simulink model "other"  (R2025a)
settings: Solver=VariableStepAuto  StartTime=0.0  StopTime=0.1  MaxStep=1e-7  RelTol=1e-3
undefined symbols (not defined in the file): Acid, Lead
libraries: spsPWMGeneratorDCDCLib x8, spsMosfetLib x4, spsCurrentMeasurementLib x3, spsSeriesRLCBranchLib x3, spsVoltageMeasurementLib x2, spsBatteryLib x1, spsDCVoltageSourceLib x1, spsGroundLib x1, spsPVArrayLib x1, spspowerguiLib x1
settings Model: Creator=GNKRISHNAN  LastModifiedBy=GNKRISHNAN

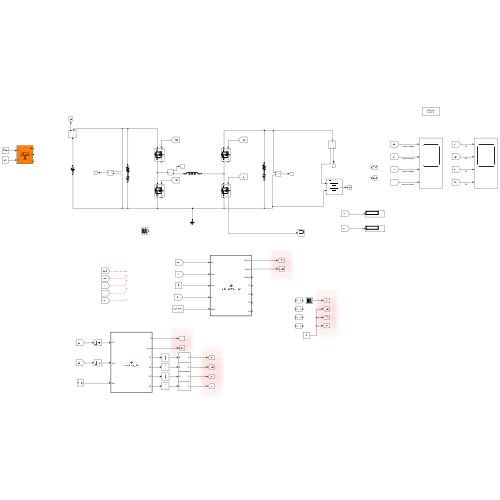
[thumbnail: Simulink's stored preview of the top-level diagram]
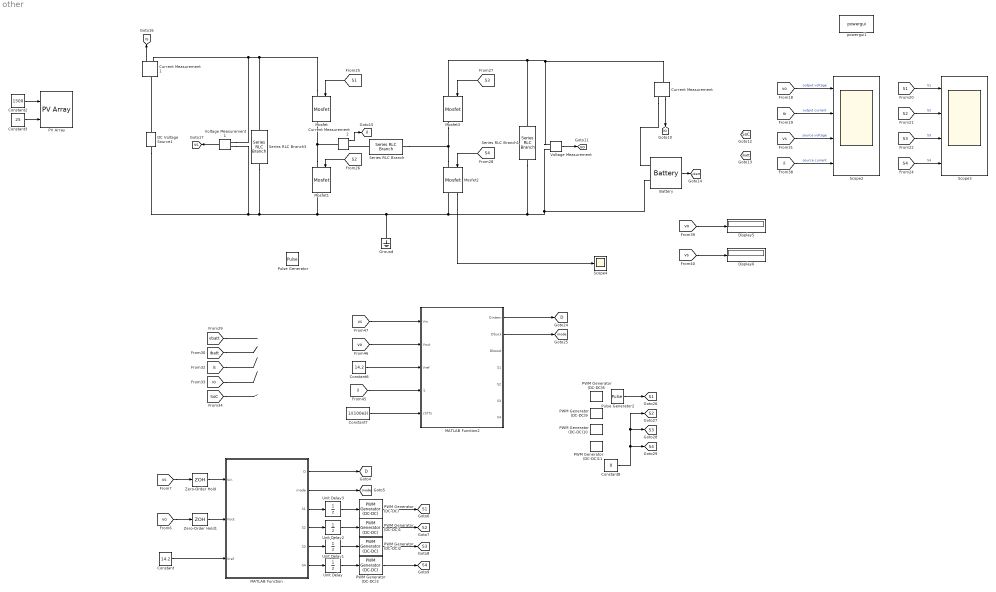
== system other ==
  Battery : spsBatteryLib/Battery  BatType=Lead-Acid  NomV=12  NomQ=5.4  SOC=80  Batt_Tr=.001  PresetModel=on  MaxQ=5.625  MinV=9  FullV=13.0658  Dis_rate=1.08  R=0.022222  Normal_OP=1.6755  expZone="[12.2171        0.018]"
  Constant : Constant  Value=14.2
  Constant2 : Constant  Value=1500
  Constant3 : Constant  Value=25
  Constant6 : Constant  Value=14.2
  Constant7 : Constant  Value=1/(100e3)
  Constant8 : Constant  Value=0
  Current Measurement : spsCurrentMeasurementLib/Current Measurement  PhasorSimulation=off  OutputType=Complex  PSBequivalent=0
  Current Measurement1 : spsCurrentMeasurementLib/Current Measurement  PhasorSimulation=off  OutputType=Complex  PSBequivalent=0
  Current Measurement2 : spsCurrentMeasurementLib/Current Measurement  PhasorSimulation=off  OutputType=Complex  PSBequivalent=0
  DC Voltage Source1 : spsDCVoltageSourceLib/DC Voltage Source  Amplitude=20  Measurements=None
  Display5 : Display
  Display6 : Display
  Ground : spsGroundLib/Ground  LConnTagsString=a
  MATLAB Function : MATLAB Function  TreatAsAtomicUnit=on  SystemSampleTime=1e-6
  MATLAB Function2 : MATLAB Function  TreatAsAtomicUnit=on  SystemSampleTime=1/(100e3)
  Mosfet{,1..3} (4 alike) : spsMosfetLib/Mosfet  Ron=0.1  Lon=0  Rd=0.0028  Vfd=0.7  IC=0  Rs=1e5  Cs=inf  Measurements=on
  PV Array : spsPVArrayLib/PV Array  Npar=1  Nser=1  PlotType=one module @ 25 deg.C & specified irradiances  S_vec="[ 1000  500  100 ]"  Temp_C_vec="[ 45 25  ]"  ModuleName=User-defined  PlotWhenSelected=off  Pm=130.032  Ncell=60  Voc=21.6  Isc=8.36  Vm=17.2  Im=7.56  beta_Voc_pc=-0.1  alpha_Isc_pc=0.001  beta_Voc=-0.0216  alpha_Isc=8.36e-05  IL=8.428  I0=1.3766e-16  nI=0.36322  Rsh=37.2573  Rs=0.33372  RobustModel=off  RobustCellTemperature=313.3991  BAL=on  Tc=1e-6  Tfilter=5e-5
  PWM Generator (DC-DC){,1..3,8..11} (8 alike) : spsPWMGeneratorDCDCLib/PWM Generator (DC-DC)  Fsw=100e3  Ts=0
  Pulse Generator : DiscretePulseGenerator  PulseType=Time based  Period=10  PulseWidth=5
  Pulse Generator2 : DiscretePulseGenerator  PulseType=Time based  Period=1/(100e3)  PulseWidth=65
  Scope2 : Scope  NumInputPorts=4
      settings: ActiveDisplayYMinimum=-3.068333797460328  ActiveDisplayYMaximum=27.615004177142961  DataLoggingVariableName=ScopeData3
  Scope3 : Scope  NumInputPorts=4
      settings: ActiveDisplayYMinimum=-0.12499999999999997  ActiveDisplayYMaximum=1.125  DataLoggingVariableName=ScopeData4
  Scope4 : Scope
      settings: ActiveDisplayYMinimum=-1.430223431644835  ActiveDisplayYMaximum=12.872010884803517  DataLoggingVariableName=ScopeData2
  Series RLC Branch : spsSeriesRLCBranchLib/Series RLC Branch  LConnTagsString=__new0  RConnTagsString=__new0  BranchType=L  Resistance=0.001  Inductance=110e-6  SetiL0=on  InitialCurrent=1  Capacitance=1e-6  Setx0=off  InitialVoltage=0  Measurements=None
  Series RLC Branch1 : spsSeriesRLCBranchLib/Series RLC Branch  LConnTagsString=__new0  RConnTagsString=__new0  BranchType=RC  Resistance=0.00001  Inductance=1e-3  SetiL0=off  InitialCurrent=0  Capacitance=120e-6  Setx0=on  InitialVoltage=12  Measurements=None
  Series RLC Branch3 : spsSeriesRLCBranchLib/Series RLC Branch  LConnTagsString=__new0  RConnTagsString=__new0  BranchType=RC  Resistance=0.0001  Inductance=1e-3  SetiL0=off  InitialCurrent=0  Capacitance=400e-6  Setx0=on  InitialVoltage=0  Measurements=None
  Unit Delay{,1..3} (4 alike) : UnitDelay  SampleTime=-1  HasFrameUpgradeWarning=on
  Voltage Measurement : spsVoltageMeasurementLib/Voltage Measurement  PhasorSimulation=off  OutputType=Complex  PSBequivalent=0
  Voltage Measurement1 : spsVoltageMeasurementLib/Voltage Measurement  PhasorSimulation=off  OutputType=Complex  PSBequivalent=0
  Zero-Order Hold : ZeroOrderHold  SampleTime=-1
  Zero-Order Hold1 : ZeroOrderHold  SampleTime=-1
  powergui1 : spspowerguiLib/powergui  Priority=1  SimulationMode=Discrete  SampleTime=1e-7  frequency=60  Iterations=50  frequencyindice=0  Pbase=100e6  ErrMax=1e-4  UnitsV=kV  UnitsW=MW  buscounter=0  FunctionMessages=off  echomessages=off  EnableUseOfTLC=off  CurrentSourceSwitches=off  DisableSnubberDevices=off  DisableRonSwitches=off  DisableVfSwitches=off  DisplayEquations=off  AutomaticDiscreteSolvers=off  SolverType=Tustin/Backward Euler (TBE)  Interpol=off  ExternalGateDelay=off  methode=off  Ts=100  x0status=blocks  SPID=on  SwTol=0  HookPort=off  NonlinearTolerance=1e-4  nMaxIteration=100  ContinueOnMaxIteration=off  RestoreLinks=warning  ResistiveCurrentMeasurement=off  Frange=[0:2:500]  Ylog=off  Xlog=on  ShowGrid=off  save=off  variable=ZData  structure=0  ZoomFFT=off  StartTime=0.0  cycles=1  DisplayStyle=1  fundamental=60  FreqAxis=off  MaxFrequency=1000  frequencyindicesteady=1  RmsSteady=1  display=off
  tag scope: D=global, S1=global, S2=global, S3=global, S4=global, SoC=global, ibatt=global, il=global, io=global, is=global, mode=global, vbatt=global, vo=global, vs=global
  wires:
  MATLAB Function/4(S2) -> Unit Delay2/1
  MATLAB Function/5(S3) -> Unit Delay1/1
  MATLAB Function/3(S1) -> Unit Delay3/1
  MATLAB Function/1(D) -> [D]
  MATLAB Function/2(mode) -> [mode]
  [vs] -> Zero-Order Hold/1
  [vo] -> Zero-Order Hold1/1
  MATLAB Function/6(S4) -> Unit Delay/1
  Constant/1 -> MATLAB Function/3(Vref)
  Zero-Order Hold/1 -> MATLAB Function/1(Vin)
  Zero-Order Hold1/1 -> MATLAB Function/2(Vout)
  PWM Generator (DC-DC)/1 -> [S1]
  PWM Generator (DC-DC)1/1 -> [S2]
  PWM Generator (DC-DC)2/1 -> [S3]
  PWM Generator (DC-DC)3/1 -> [S4]
  Unit Delay/1 -> PWM Generator (DC-DC)3/1
  Unit Delay1/1 -> PWM Generator (DC-DC)2/1
  Unit Delay2/1 -> PWM Generator (DC-DC)1/1
  Unit Delay3/1 -> PWM Generator (DC-DC)/1
  [vbatt] -> ?
  [ibatt] -> ?
  [is] -> ?
  [SoC] -> ?
  [io] -> ?
  Mosfet2/1 -> Scope4/1
  [S4] -> Scope3/4  "S4"
  [vo] -> Display5/1
  Current Measurement/1 -> [io]
  Current Measurement1/1 -> [is]
  [vs] -> Scope2/3  "source voltage"
  [S2] -> Mosfet1/1
  Voltage Measurement1/1 -> [vs]
  [S2] -> Scope3/2  "S2"
  Constant3/1 -> PV Array/2
  Voltage Measurement/1 -> [vo]
  [S1] -> Scope3/1  "S1"
  [vo] -> Scope2/1  "output voltage"
  [il] -> Scope2/4  "source current"
  [S4] -> Mosfet2/1
  [S1] -> Mosfet/1
  [S3] -> Mosfet3/1
  Current Measurement2/1 -> [il]
  [S3] -> Scope3/3  "S3"
  Battery/1 -> [vbatt]
  Constant2/1 -> PV Array/1
  [vs] -> Display6/1
  [io] -> Scope2/2  "output current"
  Constant6/1 -> MATLAB Function2/3(Vref)
  [vs] -> MATLAB Function2/1(Vin)
  MATLAB Function2/2(Dbuck) -> [mode]
  Constant7/1 -> MATLAB Function2/5(ctrlTs)
  [il] -> MATLAB Function2/4(iL)
  Pulse Generator2/1 -> [S1]
  [vo] -> MATLAB Function2/2(Vout)
  MATLAB Function2/1(Dintern) -> [D]
  Constant8/1 -> [S4], [S3], [S2]
  connections:
  Ground/LConn1 -- Mosfet1/RConn1 -- DC Voltage Source1/LConn1 -- Voltage Measurement1/LConn2 -- Series RLC Branch3/RConn1 -- Mosfet2/RConn1 -- Voltage Measurement/LConn2 -- Battery/LConn2 -- Series RLC Branch1/RConn1
  Series RLC Branch1/LConn1 -- Voltage Measurement/LConn1 -- Current Measurement/LConn1 -- Mosfet3/LConn1
  Mosfet1/LConn1 -- Current Measurement2/LConn1 -- Mosfet/RConn1
  Mosfet2/LConn1 -- Mosfet3/RConn1 -- Series RLC Branch/RConn1
  Mosfet/LConn1 -- Series RLC Branch3/LConn1 -- Current Measurement1/RConn1 -- Voltage Measurement1/LConn1
  Series RLC Branch/LConn1 -- Current Measurement2/RConn1
  DC Voltage Source1/RConn1 -- Current Measurement1/LConn1
  Current Measurement/RConn1 -- Battery/LConn1

== matlab function other/MATLAB Function ==
  data: Vin input; D output; Vout input; Vref input; mode output; S1 output; S2 output; S3 output; S4 output
function [D, mode, S1, S2, S3, S4] = controlLogic_fixed(Vin, Vout, Vref)
% Bidirectional 4-switch converter control with PI loop
% Robust startup with sensing stage before enabling switching.

% --- Parameters ---
Vhyst = 0.2;
Dmin  = 0.05;
Dmax  = 0.88;
Dinit = 0.05;
Kp = 0.01;
Ki = 0.001;
DrateLimit   = 0.005;
D_ramp_rate  = 0.0005;
softRate     = 0.01;

% Stability detector
Vtol = 0.02;             % stability tolerance
stableCountReq = 30;     % consecutive stable samples
maxSenseSamples = 5000;  % safety limit

% --- Persistent state ---
persistent lastMode integ lastD Vref_ramp controllerState ...
          Vbatt_measured stableCounter lastV sampleWindowCount
if isempty(lastMode), lastMode = -1; end
if isempty(integ), integ = 0; end
if isempty(lastD), lastD = Dinit; end
if isempty(Vref_ramp), Vref_ramp = 0; end
if isempty(controllerState), controllerState = -1; end
if isempty(Vbatt_measured), Vbatt_measured = 0; end
if isempty(stableCounter), stableCounter = 0; end
if isempty(lastV), lastV = Vout; end
if isempty(sampleWindowCount), sampleWindowCount = 0; end

% --- Init outputs ---
D   = lastD;
mode = lastMode;
S1 = 0; S2 = 0; S3 = 0; S4 = 0; % safe OFF

% --- State machine ---
switch controllerState
    case -1 % SENSE battery
        dv = abs(Vout - lastV);
        lastV = Vout;
        sampleWindowCount = sampleWindowCount + 1;

        if dv <= Vtol
            stableCounter = stableCounter + 1;
        else
            stableCounter = 0;
        end

        % Running average of battery
        if sampleWindowCount == 1
            Vbatt_measured = Vout;
        else
            Vbatt_measured = ...
                ((sampleWindowCount-1)*Vbatt_measured + Vout) / sampleWindowCount;
        end

        if stableCounter >= stableCountReq || sampleWindowCount >= maxSenseSamples
            % --- Select operating mode ---
            if (Vin >= 16+Vhyst && Vin <= 20) || (lastMode==0 && Vin > 15.5)
                mode = 0; % Buck
            elseif (Vin <= 12-Vhyst && Vin >= 8) || (lastMode==1 && Vin < 12.5)
                mode = 1; % Boost
            elseif (Vin >= 13-Vhyst && Vin <= 15+Vhyst) || lastMode==2
                mode = 2; % Buck-Boost
            else
                % fallback to battery voltage
                if Vbatt_measured > 15.5
                    mode = 0;
                elseif Vbatt_measured < 12.5
                    mode = 1;
                else
                    mode = 2;
                end
            end

            % reset control vars
            controllerState = 1; % go to ramp
            integ = 0;
            lastD = Dinit;
            Vref_ramp = 0;
        end
        D = 0;

    case 1 % DUTY_RAMP
        D_ramped = min(lastD + D_ramp_rate, Dmax);
        if Vout >= Vref
            controllerState = 2; % switch to PI
            integ = D_ramped;
            D = D_ramped;
        else
            D = D_ramped;
        end

    case 2 % PI_CONTROL
        Vref_ramp = min(Vref_ramp + softRate, Vref);
        err = Vref_ramp - Vout;
        D_commanded = Kp*err + integ;

        % Rate limit
        deltaD = D_commanded - lastD;
        deltaD_limited = max(-DrateLimit, min(DrateLimit, deltaD));
        D_unclamped = lastD + deltaD_limited;

        % Clamp
        D = max(min(D_unclamped, Dmax), Dmin);

        % Anti-windup
        if (err > 0 && D < Dmax) || (err < 0 && D > Dmin)
            integ = integ + Ki*err;
        end

    otherwise
        controllerState = -1;
        D = 0; integ = 0; Vref_ramp = 0;
        stableCounter = 0; sampleWindowCount = 0;
end

lastD = D;
lastMode = mode;

% --- Switch map ---
if controllerState <= 0
    % keep OFF during sensing
    S1 = 0; S2 = 0; S3 = 0; S4 = 0;
else
    Dbar = 1 - D;
    switch mode
        case 0 % Buck
            S1 = D;     S2 = Dbar;  S3 = 1;    S4 = 0;
        case 1 % Boost
            S1 = 1;     S2 = 0;     S3 = Dbar; S4 = D;
        case 2 % Buck-Boost
            S1 = D;     S2 = Dbar;  S3 = Dbar; S4 = D;
        otherwise
            S1 = 0; S2 = 0; S3 = 0; S4 = 0;
    end
end

end

== matlab function other/MATLAB Function2 ==
  data: Vin input; Dintern output; Vout input; Vref input; iL input; Dbuck output; Dboost output; S1 output; S2 output; S3 output; S4 output; ctrlTs input
function [Dintern, Dbuck, Dboost, S1, S2, S3, S4] = FSBB_controller_sim(Vin, Vout, Vref, iL ,ctrlTs)
% FSBB_controller_sim - cascaded voltage/current PI with Dintern mapping
% Inputs: Vin,Vout,iL,Vref,ctrlTs
% Outputs: Dintern, Dbuck, Dboost (0..1), S1..S4 boolean PWM bits (int32)
% Codegen-friendly

% Tunable params (start values)
fsw = 100e3;
Kpv = 5.0; Kiv = 25;      % outer PI (V->I)
Kpc = 0.5; Kic = 50.0;    % inner PI (I->D)
map_gain = 0.005;          % duty per amp (tune)
Dmin = 0.1; Dmax = 0.88;
Imax = 9.0;

% Persistents
persistent intV intI Dintern_last pwmPhase
if isempty(intV), intV = 0; end
if isempty(intI), intI = 0; end
if isempty(Dintern_last), Dintern_last = 1.0; end
if isempty(pwmPhase), pwmPhase = 0.0; end

% Outer PI -> Iref
Verr = Vref - Vout;
intV = intV + Kiv * ctrlTs * Verr;
Iref = Kpv * Verr + intV;
Iref = max(min(Iref, Imax*0.9), -Imax*0.9);

% Inner PI -> produce Dintern_target
Ierr = Iref - iL;
intI = intI + Kic * ctrlTs * Ierr;
u = Kpc * Ierr + intI;
Dff = 1.0;
D_target = Dff + map_gain * u;

% clamp Dintern to [0.02 1.98]
D_target = min(max(D_target, 0.02), 1.98);

% anti-windup
if (D_target <= 0.02) || (D_target >= 1.98)
    intI = intI * 0.5;
end

Dintern = D_target;
Dintern_last = Dintern;

% map Dintern to per-leg duties (paper mapping)
if Dintern <= 1.0
    Dbuck = Dintern;
    Dboost = 1.0;
else
    Dbuck = 1.0;
    Dboost = 2.0 - Dintern;
end

% clamp leg duties
Dbuck = min(max(Dbuck, Dmin), Dmax);
Dboost = min(max(Dboost, Dmin), Dmax);

% PWM phase accumulator
pwmPhase = pwmPhase + ctrlTs * fsw;
if pwmPhase >= 1.0, pwmPhase = pwmPhase - floor(pwmPhase); end

pwmBuck = (pwmPhase < Dbuck);
pwmBoost = (pwmPhase < Dboost);

% simple complementary outputs (you should insert dead-time block)
S1 = int32(pwmBuck);   % Buck high-side
S2 = int32(~pwmBuck);  % Buck low-side
S4 = int32(pwmBoost);  % Boost high-side
S3 = int32(~pwmBoost); % Boost low-side

end
